simulink model "Controller"  (R2020a)
settings: Solver=VariableStepAuto  StartTime=0.0  StopTime=10.0  RelTol=1e-3
values from neighbouring files (symbols this model uses):
  Cv = [0 0 0 0 0 1 3 5 7 9 11 14 17 21 27 34 43 57 75 91 100]    [ballvalve.m]
  deg = linspace(0,90,21)    [ballvalve.m]
  HighInit = 4500    [Simulation_Constants.m]
  Kd = 0.002    [Simulation_Constants.m]
  Ki = 1    [Simulation_Constants.m]
  Kp = 10    [Simulation_Constants.m]
  SetPres = 600    [Simulation_Constants.m]
  VHigh = 6.8/3.78    (= 1.79894179894)    [Simulation_Constants.m]
  Vinit = 4    [Simulation_Constants.m]
settings Model: Creator=twoan  LastModifiedBy=twoan
settings SolverCC: ZeroCrossAlgorithm=Adaptive
settings DebuggingCC: IgnoredZcDiagnostic=none

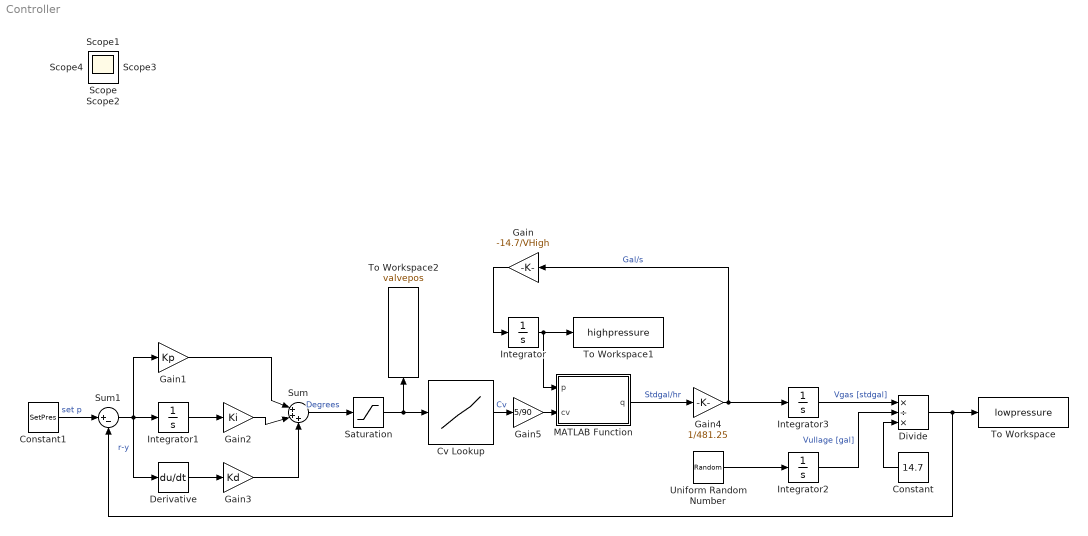
== system Controller ==
  Constant : Constant  Value=14.7
  Constant1 : Constant  Value=SetPres
  Cv Lookup : Lookup_n-D  NumberOfTableDimensions=1  BreakpointsForDimension1=deg  Table=Cv  DiagnosticForOutOfRangeInput=Warning  InternalRulePriority=Speed  RndMeth=Simplest  InputSameDT=on
  Derivative : Derivative
  Divide : Product  Inputs=*/*
  Gain : Gain  Gain=-14.7/VHigh
  Gain1 : Gain  Gain=Kp
  Gain2 : Gain  Gain=Ki
  Gain3 : Gain  Gain=Kd
  Gain4 : Gain  Gain=1/481.25
  Gain5 : Gain  Gain=5/90
  Integrator : Integrator  InitialCondition=HighInit
  Integrator1 : Integrator
  Integrator2 : Integrator  InitialCondition=0.25  LimitOutput=on  UpperSaturationLimit=Vinit
  Integrator3 : Integrator
  MATLAB Function : MATLAB Function  TreatAsAtomicUnit=on
  Saturation : Saturate  UpperLimit=90  LowerLimit=0
  Sum : Sum  Inputs=|+++
  Sum1 : Sum  Inputs=|+-
  To Workspace : ToWorkspace  VariableName=lowpressure  SaveFormat=Timeseries  SampleTime=-1
  To Workspace1 : ToWorkspace  VariableName=highpressure  SaveFormat=Timeseries  SampleTime=-1
  To Workspace2 : ToWorkspace  VariableName=valvepos  SaveFormat=Timeseries  SampleTime=-1
  Uniform Random Number : UniformRandomNumber  Minimum=0  Maximum=0.5  SampleTime=1
  Scope{,1..4} (5 alike) : Scope
  wires:
  Uniform Random Number/1 -> Integrator2/1
  Sum/1 -> Saturation/1  "Degrees"
  Cv Lookup/1 -> Gain5/1  "Cv"
  Sum1/1 -> Integrator1/1, Gain1/1, Derivative/1  "r-y"
  Integrator1/1 -> Gain2/1
  Gain2/1 -> Sum/2
  Gain1/1 -> Sum/1
  Derivative/1 -> Gain3/1
  Gain3/1 -> Sum/3
  MATLAB Function/1(q) -> Gain4/1  "Stdgal/hr"
  Integrator/1 -> MATLAB Function/1(p), To Workspace1/1
  Constant1/1 -> Sum1/1  "set p"
  Divide/1 -> To Workspace/1, Sum1/2
  Gain4/1 -> Gain/1, Integrator3/1  "Gal/s"
  Integrator2/1 -> Divide/2  "Vullage [gal]"
  Integrator3/1 -> Divide/1  "Vgas [stdgal]"
  Constant/1 -> Divide/3
  Gain/1 -> Integrator/1
  Saturation/1 -> To Workspace2/1, Cv Lookup/1
  Gain5/1 -> MATLAB Function/2(cv)

== matlab function Controller/MATLAB Function ==
  data: p input; q output; cv input
function q = fcn(p,cv)
q=cv/sqrt(520)*600*p;
end
